simulink model "frequence_response_3"  (R2021b)
settings: Solver=VariableStepAuto  StartTime=0.0  StopTime=30  RelTol=1e-3
values from neighbouring files (symbols this model uses):
  U3_max = [1 -0.25]    [main.m]    (also in main1.m = [4 6])
undefined symbols (not defined in the file or in its folder): A, B, C, D
settings Model: Creator=PaoloA  LastModifiedBy=PaoloA

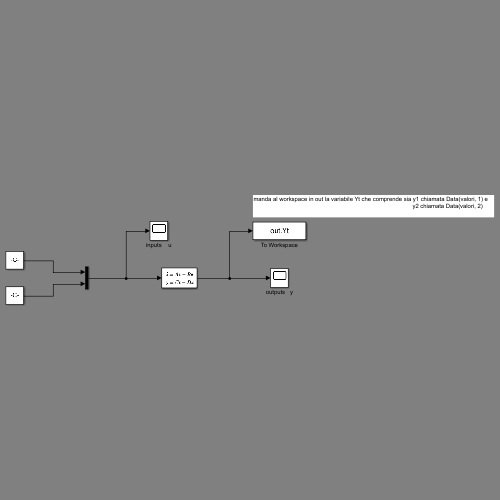
[thumbnail: Simulink's stored preview of the top-level diagram]
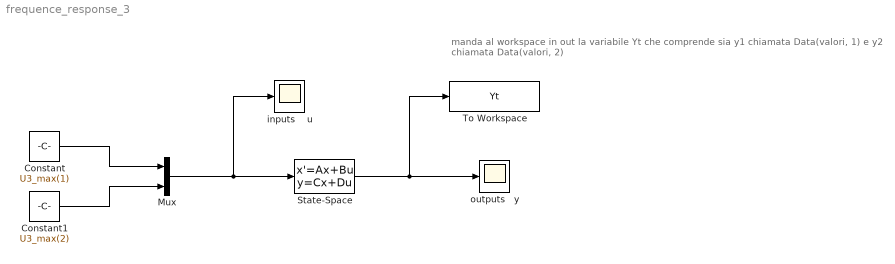
== system frequence_response_3 ==
  note: manda al workspace in out la variabile Yt che comprende sia y1 chiamata Data(valori, 1) e
      | 												           y2 chiamata Data(valori, 2)
  Constant : Constant  Value=U3_max(1)
  Constant1 : Constant  Value=U3_max(2)  VectorParams1D=off
  Mux : Mux  Inputs=2
  State-Space : StateSpace  A=A  B=B  C=C  D=D  InitialCondition=0
  To Workspace : ToWorkspace  VariableName=Yt  SaveFormat=Timeseries  SampleTime=-1
  inputs    u : Scope
  outputs   y : Scope
  wires:
  State-Space/1 -> To Workspace/1, outputs   y/1
  Mux/1 -> inputs    u/1, State-Space/1
  Constant/1 -> Mux/1
  Constant1/1 -> Mux/2
